simulink model "bpsk_rx4"  (Simulink 7.6)
settings: Solver=FixedStepDiscrete  StartTime=0.0  StopTime=1000  RelTol=1e-3
libraries: dsp_blocks x7, simulink x2
settings Model: Creator=Joshan  LastModifiedBy=Joshan

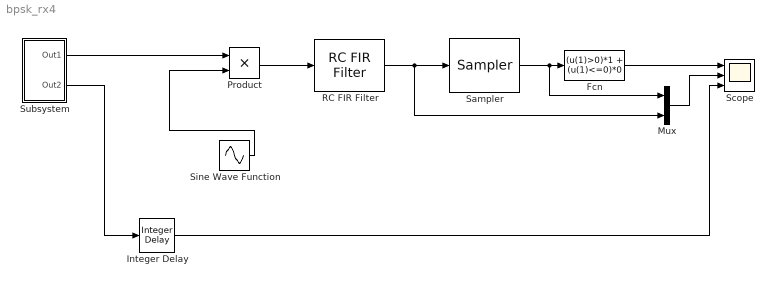
== system bpsk_rx4 ==
  Fcn : Fcn  Expr=(u(1)>0)*1 + (u(1)<=0)*0
  Integer Delay : simulink/Discrete/Integer Delay  NumDelays=256  vinit=0.0  samptime=-1
  Mux : Mux  Inputs=2
  Product : Product  RndMeth=Zero
  RC FIR Filter : dsp_blocks/Filters/RC FIR Filter  SystemSampleTime=-1  period=50  beta=0.5  root=on  filt_len=512  win_type=on
  Sampler : dsp_blocks/Conversions/Sampler  SystemSampleTime=-1  offset=80  samp_period=50
  Scope : Scope  NumInputPorts=3
      settings: YMin=-2~-2~-2  YMax=2~2~2
  Sine Wave Function : Sin  Amplitude=2  Frequency=2*pi*0.1  SampleTime=0
  Subsystem : Subsystem
  wires:
  Subsystem/1(Out1) -> Product/1
  Subsystem/2(Out2) -> Integer Delay/1
  Sine Wave Function/1 -> Product/2
  Product/1 -> RC FIR Filter/1
  RC FIR Filter/1 -> Sampler/1, Mux/2
  Fcn/1 -> Scope/1
  Mux/1 -> Scope/2
  Integer Delay/1 -> Scope/3
  Sampler/1 -> Fcn/1, Mux/1

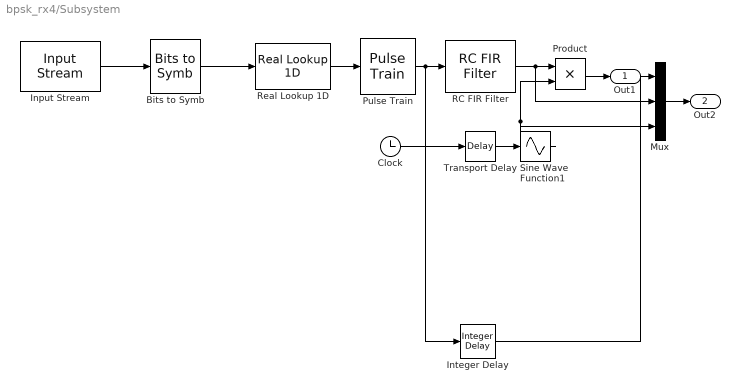
== system bpsk_rx4/Subsystem ==
  Bits to Symb : dsp_blocks/Conversions/Bits to Symb  SystemSampleTime=-1
  Clock : Clock
      settings: Decimation=10
  Input Stream : dsp_blocks/Sources//Sinks/Input Stream  SystemSampleTime=-1  period=50  width=1  fname=rand.mat
  Integer Delay : simulink/Discrete/Integer Delay  NumDelays=256  vinit=0.0  samptime=-1
  Mux : Mux  Inputs=3
  Product : Product  RndMeth=Zero
  Pulse Train : dsp_blocks/Conversions/Pulse Train  SystemSampleTime=-1  period=50
  RC FIR Filter : dsp_blocks/Filters/RC FIR Filter  SystemSampleTime=-1  period=50  beta=0.5  root=on  filt_len=512  win_type=on
  Real Lookup 1D : dsp_blocks/Conversions/Real Lookup 1D  SystemSampleTime=-1  table=[-1 1]
  Sine Wave Function1 : Sin  TimeSource=Use external signal  Frequency=2*pi*0.1  SampleTime=0
  Transport Delay : TransportDelay
  Out1 : Outport
  Out2 : Outport  Port=2
  wires:
  Bits to Symb/1 -> Real Lookup 1D/1
  Input Stream/1 -> Bits to Symb/1
  Real Lookup 1D/1 -> Pulse Train/1
  Pulse Train/1 -> RC FIR Filter/1, Integer Delay/1
  RC FIR Filter/1 -> Product/1, Mux/2
  Sine Wave Function1/1 -> Product/2, Mux/3
  Integer Delay/1 -> Mux/1
  Product/1 -> Out1/1
  Mux/1 -> Out2/1
  Clock/1 -> Transport Delay/1
  Transport Delay/1 -> Sine Wave Function1/1
